simulink model "simulation"  (R2022a)
settings: Solver=VariableStepAuto  StartTime=0.0  StopTime=150  FixedStep=1e-4  RelTol=1e-3
settings Model: Creator=me  LastModifiedBy=radek
settings DebuggingCC: UnconnectedInputMsg=warning  UnconnectedOutputMsg=warning  UnconnectedLineMsg=warning
settings RTWCC: DLArmComputeVersion=19.05

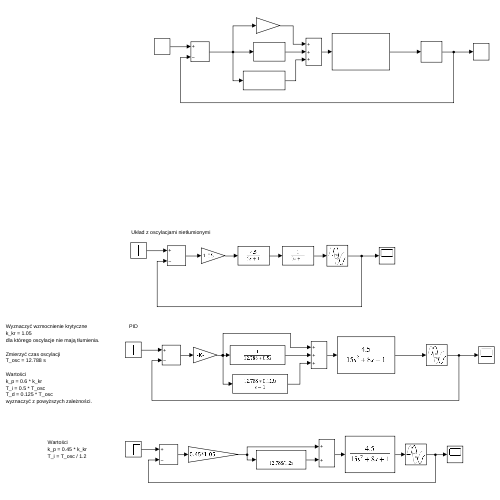
[thumbnail: Simulink's stored preview of the top-level diagram]
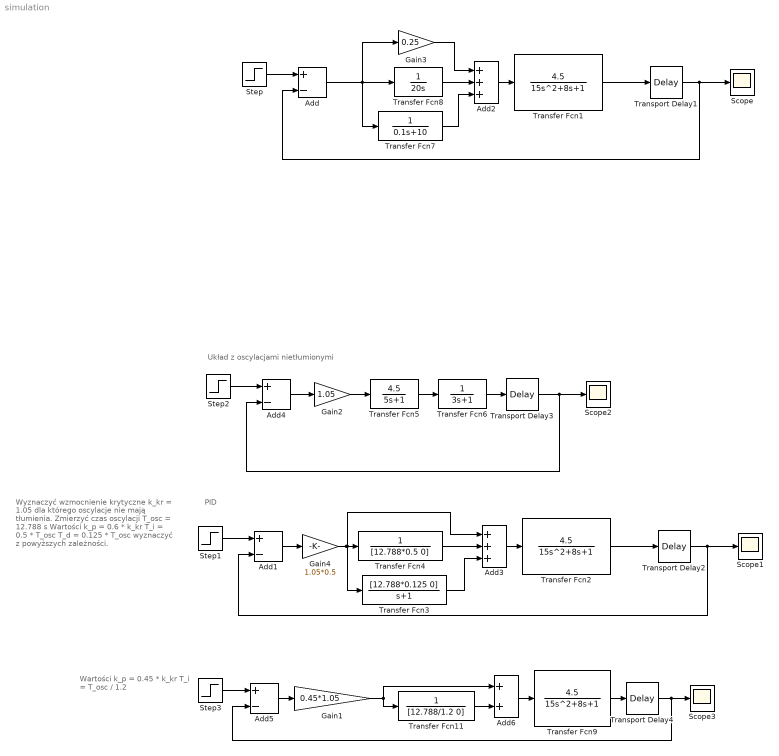
== system simulation ==
  note: PID
  note: Układ z oscylacjami nietłumionymi
  note: Wartości
      | k_p = 0.45 * k_kr
      | T_i = T_osc / 1.2
  note: Wyznaczyć wzmocnienie krytyczne
      | k_kr = 1.05
      | dla którego oscylacje nie mają tłumienia.
      |
      | Zmierzyć czas oscylacji
      | T_osc = 12.788 s
      |
      | Wartości
      | k_p = 0.6 * k_kr
      | T_i = 0.5 * T_osc
      | T_d = 0.125 * T_osc
      | wyznaczyć z powyższych zależności.
  Add{,1,4..5} (4 alike) : Sum  Inputs=+-
  Add2 : Sum  Inputs=+++
  Add3 : Sum  Inputs=+++
  Add6 : Sum
  Gain1 : Gain  Gain=0.45*1.05
  Gain2 : Gain  Gain=1.05
  Gain3 : Gain  Gain=0.25
  Gain4 : Gain  Gain=1.05*0.5
  Scope{,1..3} (4 alike) : Scope
  Step{,1..3} (4 alike) : Step  Time=0  SampleTime=0
  Transfer Fcn1 : TransferFcn  Numerator=4.5  Denominator=[15 8 1]
  Transfer Fcn11 : TransferFcn  Denominator=[12.788/1.2 0]
  Transfer Fcn2 : TransferFcn  Numerator=4.5  Denominator=[15 8 1]
  Transfer Fcn3 : TransferFcn  Numerator=[12.788*0.125 0]  Denominator=[1 1]
  Transfer Fcn4 : TransferFcn  Denominator=[12.788*0.5 0]
  Transfer Fcn5 : TransferFcn  Numerator=[4.5]  Denominator=[5 1]
  Transfer Fcn6 : TransferFcn  Denominator=[3 1]
  Transfer Fcn7 : TransferFcn  Denominator=[0.1 10]
  Transfer Fcn8 : TransferFcn  Denominator=[20 0]
  Transfer Fcn9 : TransferFcn  Numerator=4.5  Denominator=[15 8 1]
  Transport Delay{1..4} (4 alike) : TransportDelay  DelayTime=2
  wires:
  Add2/1 -> Transfer Fcn1/1
  Step/1 -> Add/1
  Gain3/1 -> Add2/1
  Transfer Fcn7/1 -> Add2/3
  Transfer Fcn8/1 -> Add2/2
  Add/1 -> Transfer Fcn8/1, Transfer Fcn7/1, Gain3/1
  Transfer Fcn1/1 -> Transport Delay1/1
  Transport Delay1/1 -> Add/2, Scope/1
  Add4/1 -> Gain2/1
  Step2/1 -> Add4/1
  Transfer Fcn5/1 -> Transfer Fcn6/1
  Transfer Fcn6/1 -> Transport Delay3/1
  Transport Delay3/1 -> Add4/2, Scope2/1
  Add3/1 -> Transfer Fcn2/1
  Transfer Fcn4/1 -> Add3/2
  Transfer Fcn2/1 -> Transport Delay2/1
  Step1/1 -> Add1/1
  Transfer Fcn3/1 -> Add3/3
  Gain2/1 -> Transfer Fcn5/1
  Add1/1 -> Gain4/1
  Gain4/1 -> Add3/1, Transfer Fcn3/1, Transfer Fcn4/1
  Add6/1 -> Transfer Fcn9/1
  Transport Delay4/1 -> Scope3/1, Add5/2
  Transfer Fcn9/1 -> Transport Delay4/1
  Transfer Fcn11/1 -> Add6/2
  Add5/1 -> Gain1/1
  Gain1/1 -> Transfer Fcn11/1, Add6/1
  Step3/1 -> Add5/1
  Transport Delay2/1 -> Scope1/1, Add1/2
